simulink model "b"  (R2018b)
settings: Solver=FixedStepAuto  StartTime=0.0  StopTime=10.68  FixedStep=0.01  RelTol=1e-3
settings Model: Creator=yizha  LastModifiedBy=yizha

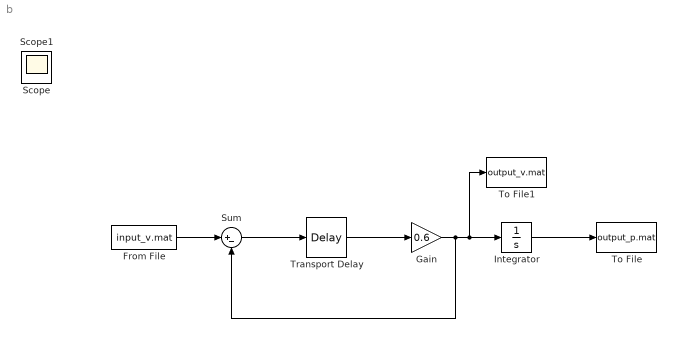
== system b ==
  From File : FromFile  FileName=input_v.mat  SampleTime=0
  Gain : Gain  Gain=0.6
  Integrator : Integrator
  Sum : Sum  Inputs=|+-
  To File : ToFile  Filename=output_p.mat
  To File1 : ToFile  Filename=output_v.mat
  Transport Delay : TransportDelay  DelayTime=0.1
  Scope : Scope
  Scope1 : Scope
  wires:
  From File/1 -> Sum/1
  Sum/1 -> Transport Delay/1
  Transport Delay/1 -> Gain/1
  Gain/1 -> To File1/1, Integrator/1, Sum/2
  Integrator/1 -> To File/1
